simulink model "CounterModel"  (R2024b)
settings: Solver=VariableStepAuto  StartTime=0.0  StopTime=10.0  RelTol=1e-3
settings Model: Creator=Ahmad  LastModifiedBy=Ahmad

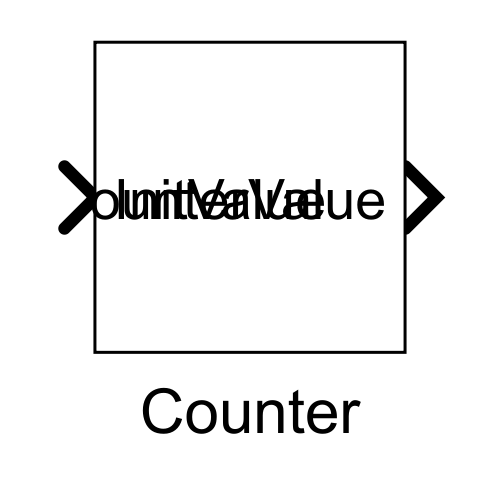
[thumbnail: Simulink's stored preview of the top-level diagram]
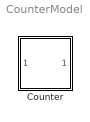
== system CounterModel ==
  Counter : Subsystem

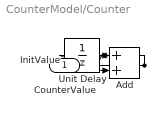
== system CounterModel/Counter ==
  InitValue : Inport
  Add : Sum
  Unit Delay : UnitDelay  SampleTime=-1  HasFrameUpgradeWarning=on
  CounterValue : Outport
  wires:
  InitValue/1 -> Add/1
  Add/1 -> CounterValue/1, Unit Delay/1
  Unit Delay/1 -> Add/2
